simulink model "Project_work_simulink_2019aa"  (R2019a)
settings: Solver=VariableStepAuto  StartTime=0.0  StopTime=100  RelTol=1e-3
values from neighbouring files (symbols this model uses):
  A = (m_t/2+m_tr+m_ts)*l_t    (= 0.0946875)    [AllParameters.m]
  B = (m_m/2+m_mr+m_ms)*l_m    (= 0.11046)    [AllParameters.m]
  C = (m_b/2*l_b+m_cb*l_cb)    (= 0.02054)    [AllParameters.m]
  D = (m_b/3*l_b^2+m_cb*l_cb^2)    (= 0.00509253333333)    [AllParameters.m]
  E = (m_m/3+m_mr+m_ms)*l_m^2+(m_t/3+m_tr+m_ts)*l_t^2    (= 0.0498816166667)    [AllParameters.m]
  F = m_ms*r_ms^2+m_ts/2*r_ts^2    (= 0.006230625)    [AllParameters.m]
  g = 9.81    [AllParameters.m]
  J_mr = 2.65e-5    (= 2.65e-05)    [AllParameters.m]
  J_tr = 1.654e-5    (= 1.654e-05)    [AllParameters.m]
  J_v = Jv1+Jv2+Jv3+Jv4+Jv5+Jv6+Jv7+Jv8    (= 0.0593269625)    [AllParameters.m]
  K2 = K(:,1:end-2)    [Linear_model_control.m]
  k_h = 0.0095    [AllParameters.m]
  k_v = 0.00545    [AllParameters.m]
  Ki = K(:,7:end)    [Linear_model_control.m]
  l_b = 0.26    [AllParameters.m]
  l_m = 0.24    [AllParameters.m]
  l_t = 0.25    [AllParameters.m]
  Tm = 0.8921    [AllParameters.m]    (also in Parametrit.m)
  Ts = 10 * 10^(-3)    (= 0.01)    [Linear_model_control.m]
  Tt = 0.3423    [AllParameters.m]    (also in Parametrit.m)
undefined symbols (not defined in the file or in its folder): Cd, Gamma, Ko, Phi, polynom
libraries: simulink_extras x4
settings Model: Creator=jerek  LastModifiedBy=jerek

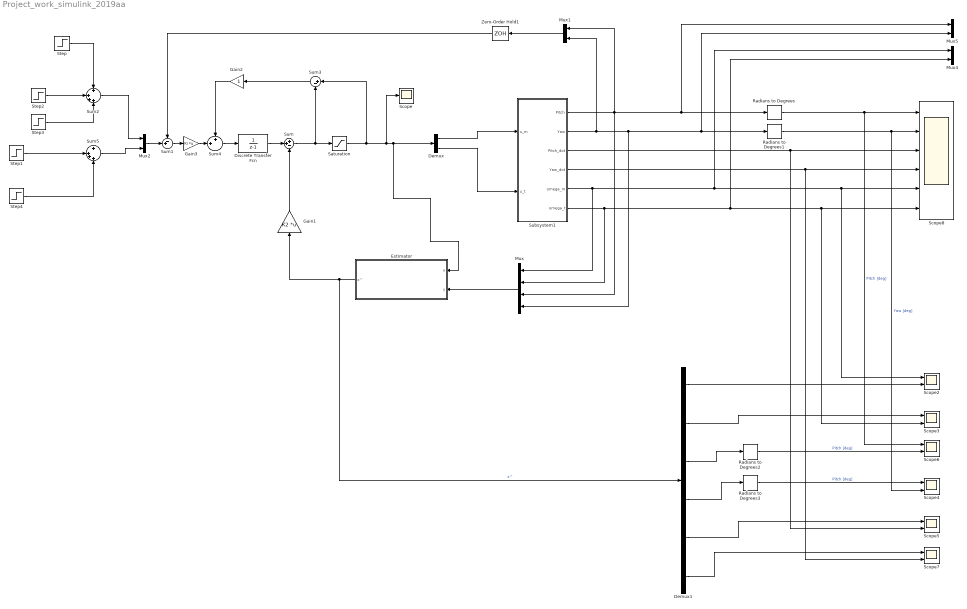
== system Project_work_simulink_2019aa ==
  Demux : Demux  Outputs=2
  Demux1 : Demux  Outputs=6
  Discrete Transfer Fcn : DiscreteTransferFcn  Denominator=[1 -1]  SampleTime=Ts
  Estimator : Subsystem
  Gain1 : Gain  Gain=K2  Multiplication=Matrix(K*u) (u vector)
  Gain2 : Gain
  Gain3 : Gain  Gain=Ki  Multiplication=Matrix(K*u) (u vector)
  Mux : Mux
  Mux{1..2,4..5} (4 alike) : Mux  Inputs=2
  Radians to Degrees{,1..3} (4 alike) : simulink_extras/Transformations/Radians to Degrees
  Saturation : Saturate  UpperLimit=18  LowerLimit=-18
  Scope : Scope
  Scope{2..7} (6 alike) : Scope  NumInputPorts=2
  Scope8 : Scope  NumInputPorts=6
  Step : Step  Time=0  After=deg2rad(-5)  SampleTime=0
  Step1 : Step  Time=0  After=deg2rad(45)  SampleTime=0
  Step2 : Step  Time=15  After=deg2rad(-10)  SampleTime=0
  Step3 : Step  Time=40  After=deg2rad(-15)  SampleTime=0
  Step4 : Step  Time=30  After=deg2rad(-10)  SampleTime=0
  Subsystem1 : Subsystem
  Sum : Sum  Inputs=++-
  Sum1 : Sum  Inputs=-+|
  Sum2 : Sum  Inputs=+|+++
  Sum3 : Sum  Inputs=|+-
  Sum4 : Sum  Inputs=++|
  Sum5 : Sum  Inputs=+|+++
  Zero-Order Hold1 : ZeroOrderHold  SampleTime=Ts
  wires:
  Radians to Degrees1/1 -> Scope8/2, Scope4/2  "Yaw [deg]"
  Radians to Degrees/1 -> Scope8/1, Scope6/1  "Pitch [deg]"
  Demux/2 -> Subsystem1/2(u_t)
  Demux/1 -> Subsystem1/1(u_m)
  Mux2/1 -> Sum1/2
  Mux1/1 -> Zero-Order Hold1/1
  Subsystem1/1(Pitch) -> Mux5/1, Radians to Degrees/1, Mux/3, Mux1/1
  Subsystem1/2(Yaw) -> Mux5/2, Radians to Degrees1/1, Mux/4, Mux1/2
  Subsystem1/3(Pitch_dot) -> Scope8/3, Scope5/2
  Subsystem1/4(Yaw_dot) -> Scope8/4, Scope7/2
  Subsystem1/5(omega_m) -> Mux/1, Mux4/1, Scope8/5, Scope2/1
  Subsystem1/6(omega_t) -> Mux/2, Mux4/2, Scope8/6, Scope3/2
  Zero-Order Hold1/1 -> Sum1/1
  Demux1/1 -> Scope2/2
  Demux1/2 -> Scope3/1
  Demux1/3 -> Radians to Degrees2/1
  Radians to Degrees2/1 -> Scope6/2  "Pitch [deg]"
  Demux1/4 -> Radians to Degrees3/1
  Radians to Degrees3/1 -> Scope4/1  "Pitch [deg]"
  Demux1/5 -> Scope5/1
  Demux1/6 -> Scope7/1
  Sum/1 -> Saturation/1, Sum3/2
  Estimator/1(x^) -> Demux1/1, Gain1/1  "x^"
  Step/1 -> Sum2/1
  Sum2/1 -> Mux2/1
  Step2/1 -> Sum2/2
  Discrete Transfer Fcn/1 -> Sum/2
  Gain1/1 -> Sum/3
  Sum4/1 -> Discrete Transfer Fcn/1
  Step1/1 -> Sum5/2
  Step4/1 -> Sum5/4
  Sum5/1 -> Mux2/2
  Sum1/1 -> Gain3/1
  Gain3/1 -> Sum4/2
  Gain2/1 -> Sum4/1
  Sum3/1 -> Gain2/1
  Saturation/1 -> Sum3/1, Scope/1, Estimator/1(u), Demux/1
  Mux/1 -> Estimator/2(y)
  Step3/1 -> Sum2/4

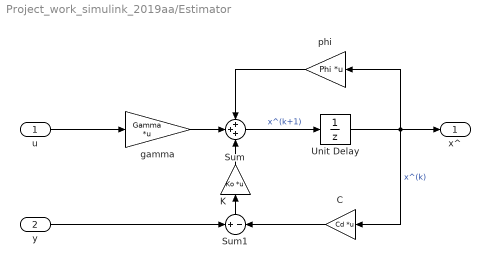
== system Project_work_simulink_2019aa/Estimator ==
  u : Inport
  y : Inport  Port=2
  C : Gain  Gain=Cd  Multiplication=Matrix(K*u)  SaturateOnIntegerOverflow=on  OutDataTypeStr=Inherit: Same as input  ParamDataTypeStr=Inherit: Same as input
  K : Gain  Gain=Ko  Multiplication=Matrix(K*u)  SaturateOnIntegerOverflow=on  OutDataTypeStr=Inherit: Same as input  ParamDataTypeStr=Inherit: Same as input
  Sum : Sum  Inputs=+++  SaturateOnIntegerOverflow=on
  Sum1 : Sum  Inputs=+-  SaturateOnIntegerOverflow=on
  Unit Delay : UnitDelay  SampleTime=Ts
  gamma : Gain  Gain=Gamma  Multiplication=Matrix(K*u)  SaturateOnIntegerOverflow=on  OutDataTypeStr=Inherit: Same as input  ParamDataTypeStr=Inherit: Same as input
  phi : Gain  Gain=Phi  Multiplication=Matrix(K*u)  SaturateOnIntegerOverflow=on  OutDataTypeStr=Inherit: Same as input  ParamDataTypeStr=Inherit: Same as input
  x^ : Outport
  wires:
  u/1 -> gamma/1
  Sum/1 -> Unit Delay/1  "x^(k+1)"
  Unit Delay/1 -> phi/1, x^/1, C/1  "x^(k)"
  phi/1 -> Sum/1
  gamma/1 -> Sum/2
  Sum1/1 -> K/1
  y/1 -> Sum1/1
  C/1 -> Sum1/2
  K/1 -> Sum/3

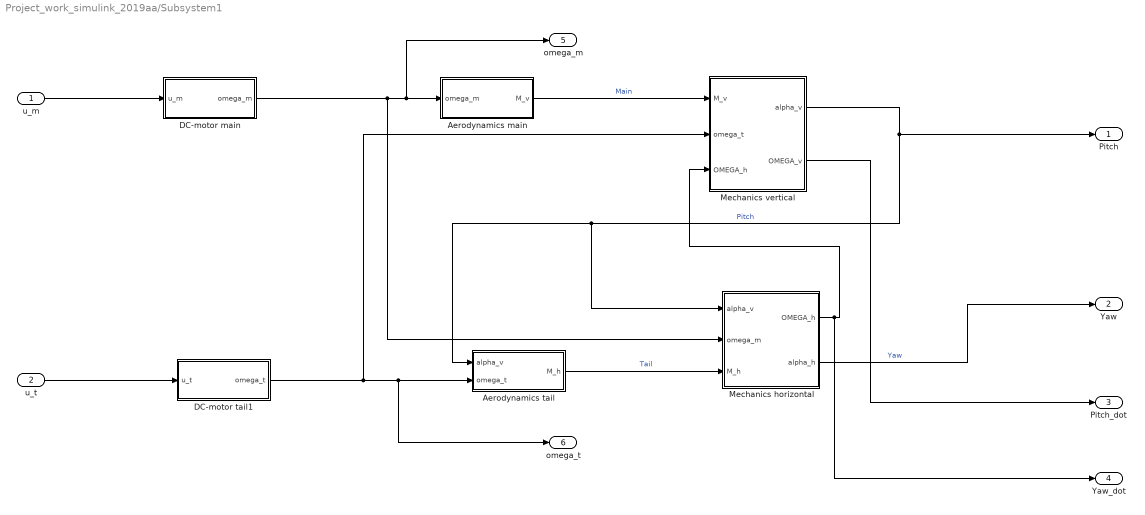
== system Project_work_simulink_2019aa/Subsystem1 ==
  u_m : Inport
  u_t : Inport  Port=2
  Aerodynamics main : Subsystem
  Aerodynamics tail : Subsystem
  DC-motor main : Subsystem
  DC-motor tail1 : Subsystem
  Mechanics horizontal : Subsystem
  Mechanics vertical : Subsystem
  Pitch : Outport
  Yaw : Outport  Port=2
  Pitch_dot : Outport  Port=3
  Yaw_dot : Outport  Port=4
  omega_m : Outport  Port=5
  omega_t : Outport  Port=6
  wires:
  DC-motor main/1(omega_m) -> Mechanics horizontal/2(omega_m), omega_m/1, Aerodynamics main/1(omega_m)
  DC-motor tail1/1(omega_t) -> Mechanics vertical/2(omega_t), omega_t/1, Aerodynamics tail/2(omega_t)
  Mechanics vertical/1(alpha_v) -> Pitch/1, Mechanics horizontal/1(alpha_v), Aerodynamics tail/1(alpha_v)  "Pitch"
  Aerodynamics tail/1(M_h) -> Mechanics horizontal/3(M_h)  "Tail"
  Mechanics horizontal/1(OMEGA_h) -> Yaw_dot/1, Mechanics vertical/3(OMEGA_h)
  Aerodynamics main/1(M_v) -> Mechanics vertical/1(M_v)  "Main"
  u_m/1 -> DC-motor main/1(u_m)
  u_t/1 -> DC-motor tail1/1(u_t)
  Mechanics horizontal/2(alpha_h) -> Yaw/1  "Yaw"
  Mechanics vertical/2(OMEGA_v) -> Pitch_dot/1

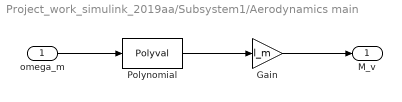
== system Project_work_simulink_2019aa/Subsystem1/Aerodynamics main ==
  omega_m : Inport
  Gain : Gain  Gain=l_m
  Polynomial : Polyval  Coefs=polynom.MainForce
  M_v : Outport  VectorParamsAs1DForOutWhenUnconnected=off
  wires:
  Polynomial/1 -> Gain/1
  Gain/1 -> M_v/1
  omega_m/1 -> Polynomial/1

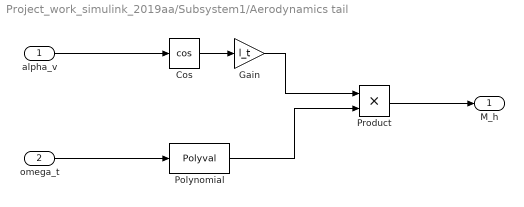
== system Project_work_simulink_2019aa/Subsystem1/Aerodynamics tail ==
  alpha_v : Inport
  omega_t : Inport  Port=2
  Cos : Trigonometry  Operator=cos
  Gain : Gain  Gain=l_t
  Polynomial : Polyval  Coefs=polynom.TailForce
  Product : Product
  M_h : Outport  VectorParamsAs1DForOutWhenUnconnected=off
  wires:
  omega_t/1 -> Polynomial/1
  alpha_v/1 -> Cos/1
  Cos/1 -> Gain/1
  Polynomial/1 -> Product/2
  Gain/1 -> Product/1
  Product/1 -> M_h/1

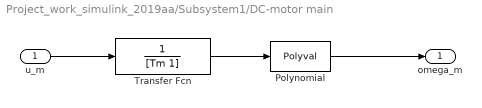
== system Project_work_simulink_2019aa/Subsystem1/DC-motor main ==
  u_m : Inport
  Polynomial : Polyval  Coefs=polynom.MainSpeed
  Transfer Fcn : TransferFcn  Denominator=[Tm 1]
  omega_m : Outport  VectorParamsAs1DForOutWhenUnconnected=off
  wires:
  Transfer Fcn/1 -> Polynomial/1
  Polynomial/1 -> omega_m/1
  u_m/1 -> Transfer Fcn/1

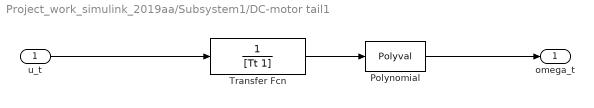
== system Project_work_simulink_2019aa/Subsystem1/DC-motor tail1 ==
  u_t : Inport
  Polynomial : Polyval  Coefs=polynom.TailSpeed
  Transfer Fcn : TransferFcn  Denominator=[Tt 1]
  omega_t : Outport  VectorParamsAs1DForOutWhenUnconnected=off
  wires:
  u_t/1 -> Transfer Fcn/1
  Polynomial/1 -> omega_t/1
  Transfer Fcn/1 -> Polynomial/1

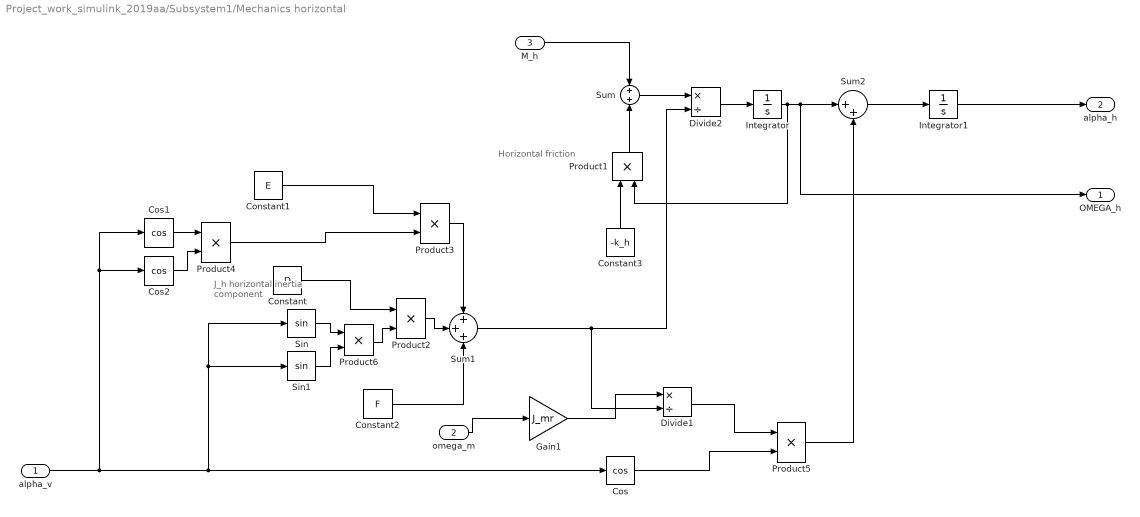
== system Project_work_simulink_2019aa/Subsystem1/Mechanics horizontal ==
  note: Horizontal friction
  note: J_h
      | horizontal inertia component
  alpha_v : Inport
  omega_m : Inport  Port=2
  M_h : Inport  Port=3
  Constant : Constant  Value=D
  Constant1 : Constant  Value=E
  Constant2 : Constant  Value=F
  Constant3 : Constant  Value=-k_h
  Cos : Trigonometry  Operator=cos
  Cos1 : Trigonometry  Operator=cos
  Cos2 : Trigonometry  Operator=cos
  Divide1 : Product  Inputs=*/
  Divide2 : Product  Inputs=*/
  Gain1 : Gain  Gain=J_mr
  Integrator : Integrator
  Integrator1 : Integrator
  Product{1..6} (6 alike) : Product
  Sin : Trigonometry
  Sin1 : Trigonometry
  Sum : Sum  Inputs=+|+
  Sum1 : Sum  Inputs=+++
  Sum2 : Sum  Inputs=|++
  OMEGA_h : Outport  VectorParamsAs1DForOutWhenUnconnected=off
  alpha_h : Outport  Port=2  VectorParamsAs1DForOutWhenUnconnected=off
  wires:
  Integrator/1 -> OMEGA_h/1, Sum2/1, Product1/2
  M_h/1 -> Sum/1
  Integrator1/1 -> alpha_h/1
  omega_m/1 -> Gain1/1
  Product5/1 -> Sum2/2
  alpha_v/1 -> Cos/1, Sin1/1, Sin/1, Cos2/1, Cos1/1
  Cos/1 -> Product5/2
  Product2/1 -> Sum1/2
  Constant/1 -> Product2/1
  Constant1/1 -> Product3/1
  Product3/1 -> Sum1/1
  Constant2/1 -> Sum1/3
  Cos1/1 -> Product4/1
  Cos2/1 -> Product4/2
  Product4/1 -> Product3/2
  Sin1/1 -> Product6/2
  Sin/1 -> Product6/1
  Product6/1 -> Product2/2
  Sum2/1 -> Integrator1/1
  Sum1/1 -> Divide2/2, Divide1/2
  Divide1/1 -> Product5/1
  Gain1/1 -> Divide1/1
  Constant3/1 -> Product1/1
  Product1/1 -> Sum/2
  Divide2/1 -> Integrator/1
  Sum/1 -> Divide2/1

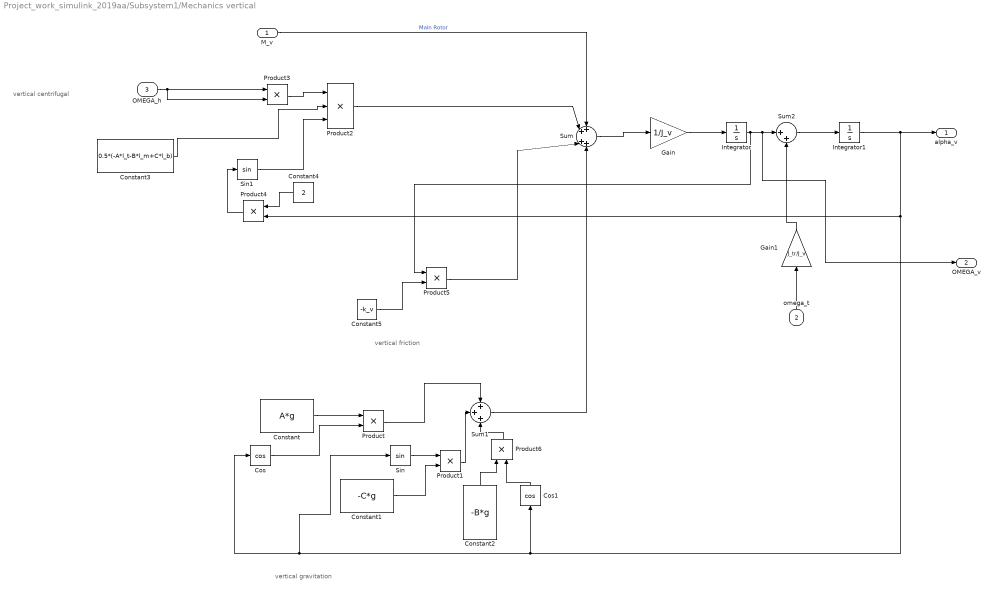
== system Project_work_simulink_2019aa/Subsystem1/Mechanics vertical ==
  note: vertical gravitation
  note: vertical friction
  note: vertical centrifugal
  M_v : Inport
  omega_t : Inport  Port=2
  OMEGA_h : Inport  Port=3
  Constant : Constant  Value=A*g
  Constant1 : Constant  Value=-C*g
  Constant2 : Constant  Value=-B*g
  Constant3 : Constant  Value=0.5*(-A*l_t-B*l_m+C*l_b)
  Constant4 : Constant  Value=2
  Constant5 : Constant  Value=-k_v
  Cos : Trigonometry  Operator=cos
  Cos1 : Trigonometry  Operator=cos
  Gain : Gain  Gain=1/J_v
  Gain1 : Gain  Gain=J_tr/J_v
  Integrator : Integrator
  Integrator1 : Integrator  InitialCondition=deg2rad(-37)
  Product{,1,3..6} (6 alike) : Product
  Product2 : Product  Inputs=3
  Sin : Trigonometry
  Sin1 : Trigonometry
  Sum : Sum  Inputs=++|++
  Sum1 : Sum  Inputs=+++
  Sum2 : Sum  Inputs=|++
  alpha_v : Outport  VectorParamsAs1DForOutWhenUnconnected=off
  OMEGA_v : Outport  Port=2  VectorParamsAs1DForOutWhenUnconnected=off
  wires:
  Integrator1/1 -> Cos1/1, Sin/1, Cos/1, Product4/2, alpha_v/1
  Sum/1 -> Gain/1
  Gain/1 -> Integrator/1
  Cos/1 -> Product/2
  Constant/1 -> Product/1
  Product/1 -> Sum1/1
  Sin/1 -> Product1/1
  Product1/1 -> Sum1/2
  Sum1/1 -> Sum/4
  Constant1/1 -> Product1/2
  M_v/1 -> Sum/1  "Main Rotor"
  OMEGA_h/1 -> Product3/2, Product3/1
  Product3/1 -> Product2/1
  Constant3/1 -> Product2/2
  Product4/1 -> Sin1/1
  Constant4/1 -> Product4/1
  Sin1/1 -> Product2/3
  Product2/1 -> Sum/2
  Integrator/1 -> OMEGA_v/1, Sum2/1, Product5/1
  Sum2/1 -> Integrator1/1
  Gain1/1 -> Sum2/2
  omega_t/1 -> Gain1/1
  Constant5/1 -> Product5/2
  Product5/1 -> Sum/3
  Cos1/1 -> Product6/2
  Product6/1 -> Sum1/3
  Constant2/1 -> Product6/1
